simulink model "alapotteresiranyitasBecslesekkelSimulink"  (R2023b)
settings: Solver=VariableStepAuto  StartTime=0.0  StopTime=100  RelTol=1e-3
values from neighbouring files (symbols this model uses):
  A = [2 5 2.3; 1 0 3; 0 -4.1 5]    [elso_ora.m]    (also in laborXI.m = [0 1;-k/m -b/m])
  B = [1;-1;-2]    [elso_ora.m]    (also in laborXI.m = [0;1/m])
  C = [-1 -2 3]    [elso_ora.m]    (also in laborXI.m = [1 0])
  G = acker(A',C',[so1 so2])'    [laborXI.m]
  K = acker(A,B,[sc1 sc2])    [laborXI.m]
  Mu = Mxu(3)    [laborXI.m]
  Mx = Mxu(1:2)    [laborXI.m]
settings Model: Creator=lenovo  LastModifiedBy=lenovo

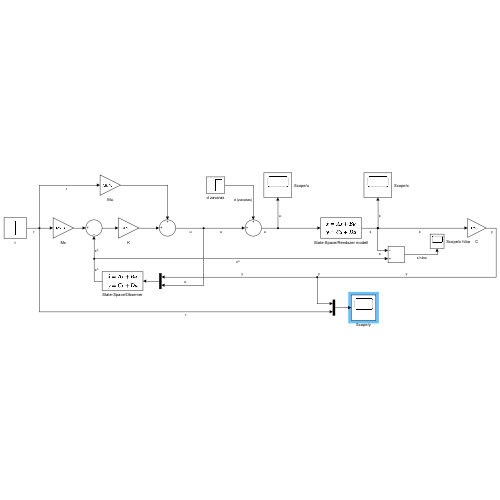
[thumbnail: Simulink's stored preview of the top-level diagram]
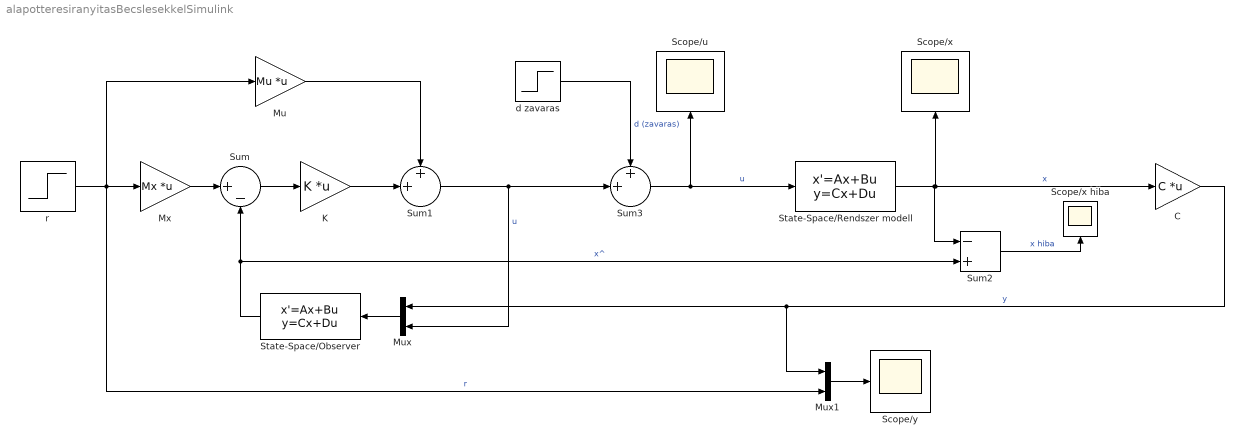
== system alapotteresiranyitasBecslesekkelSimulink ==
  C : Gain  Gain=C  Multiplication=Matrix(K*u)
  K : Gain  Gain=K  Multiplication=Matrix(K*u)
  Mu : Gain  Gain=Mu  Multiplication=Matrix(K*u)
  Mux : Mux  Inputs=2
  Mux1 : Mux  Inputs=2
  Mx : Gain  Gain=Mx  Multiplication=Matrix(K*u)
  Scope/u : Scope
  Scope/x : Scope
  Scope/x hiba : Scope
  Scope/y : Scope
  State-Space/Observer : StateSpace  A=A-G*C  B=[G B]  C=eye(2)  D=zeros(2,2)  InitialCondition=0
  State-Space/Rendszer modell : StateSpace  A=A  B=B  C=eye(2)  D=zeros(2,1)  InitialCondition=[0.1 0]
  Sum : Sum  Inputs=|+-
  Sum1 : Sum  Inputs=++|
  Sum2 : Sum  Inputs=-+
  Sum3 : Sum  Inputs=++|
  d zavaras : Step  Time=0  After=0  SampleTime=0
  r : Step  Time=40  SampleTime=0
  wires:
  State-Space/Observer/1 -> Sum/2, Sum2/2  "x^"
  State-Space/Rendszer modell/1 -> Scope/x/1, C/1, Sum2/1  "x"
  r/1 -> Mu/1, Mux1/2, Mx/1  "r"
  Mu/1 -> Sum1/1
  Mx/1 -> Sum/1
  K/1 -> Sum1/2
  Sum1/1 -> Sum3/2, Mux/2  "u"
  Sum/1 -> K/1
  C/1 -> Mux1/1, Mux/1  "y"
  Mux/1 -> State-Space/Observer/1
  Mux1/1 -> Scope/y/1
  Sum2/1 -> Scope/x hiba/1  "x hiba"
  Sum3/1 -> State-Space/Rendszer modell/1, Scope/u/1  "u"
  d zavaras/1 -> Sum3/1  "d (zavaras)"
